simulink model "waypoint_follow"  (R2024a)
settings: Solver=VariableStepAuto  StartTime=0.0  StopTime=inf  RelTol=1e-3
libraries: rllib x1
settings Model: Creator=gaura  LastModifiedBy=gaura

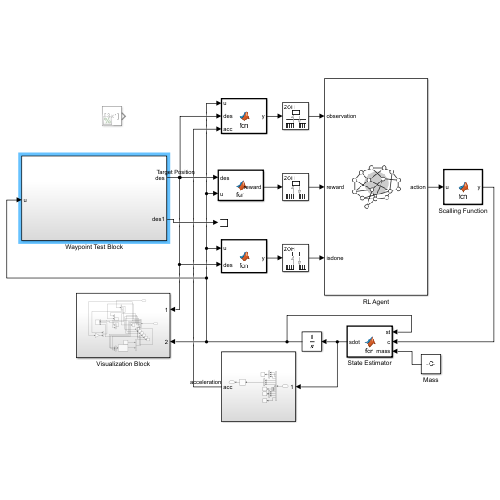
[thumbnail: Simulink's stored preview of the top-level diagram]
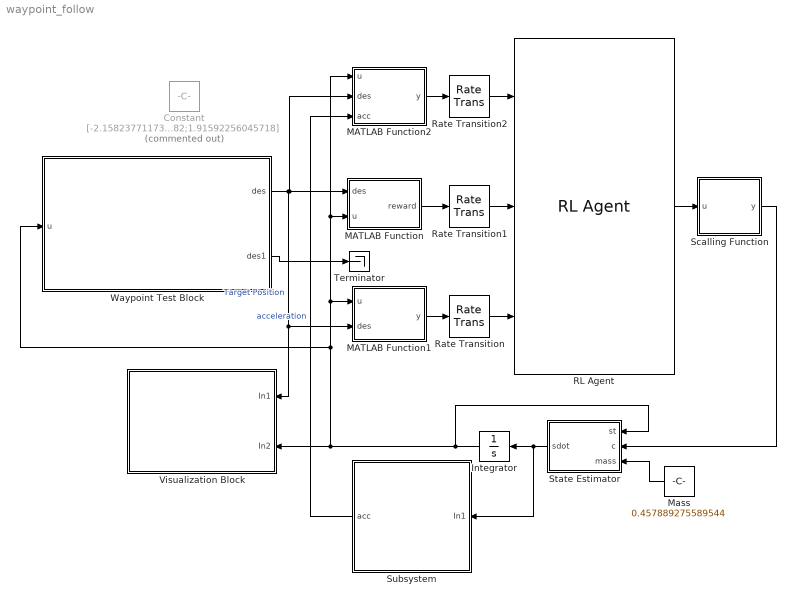
== system waypoint_follow ==
  Constant : Constant  Commented=on  Value=[-2.15823771173935;0.736471979161082;1.91592256045718]  SampleTime=-1
  Integrator : Integrator  InitialCondition=[2;-3;-1;0;0;0;0;0;0;0;0;0;0]
  MATLAB Function : MATLAB Function  TreatAsAtomicUnit=on
  MATLAB Function1 : MATLAB Function  TreatAsAtomicUnit=on
  MATLAB Function2 : MATLAB Function  TreatAsAtomicUnit=on
  Mass : Constant  Value=0.457889275589544  SampleTime=-1
  RL Agent : rllib/RL Agent  Agent=agent  ExternalActionAsInput=off  ProvideLastAction=off  ProvideCumRwd=off  TreatAsDirectFeedthrough=on  UseStrictObservationDataTypes=off
  Rate Transition : RateTransition
  Rate Transition1 : RateTransition
  Rate Transition2 : RateTransition
  Scalling Function : MATLAB Function  TreatAsAtomicUnit=on
  State Estimator : MATLAB Function  TreatAsAtomicUnit=on
  Subsystem : Subsystem
  Terminator : Terminator
  Visualization Block : Subsystem
  Waypoint Test Block : Subsystem
  wires:
  MATLAB Function/1(reward) -> Rate Transition1/1
  MATLAB Function1/1(y) -> Rate Transition/1
  MATLAB Function2/1(y) -> Rate Transition2/1
  RL Agent/1 -> Scalling Function/1(u)
  Scalling Function/1(y) -> State Estimator/2(c)
  State Estimator/1(sdot) -> Subsystem/1(In1), Integrator/1
  Integrator/1 -> MATLAB Function2/1(u), MATLAB Function/2(u), MATLAB Function1/1(u), Waypoint Test Block/1(u), Visualization Block/2(In2), State Estimator/1(st)
  Waypoint Test Block/1(des) -> MATLAB Function2/2(des), MATLAB Function/1(des), Visualization Block/1(In1), MATLAB Function1/2(des)  "Target Position"
  Rate Transition/1 -> RL Agent/3
  Rate Transition1/1 -> RL Agent/2
  Rate Transition2/1 -> RL Agent/1
  Mass/1 -> State Estimator/3(mass)
  Subsystem/1(acc) -> MATLAB Function2/3(acc)  "acceleration"
  Waypoint Test Block/2(des1) -> Terminator/1

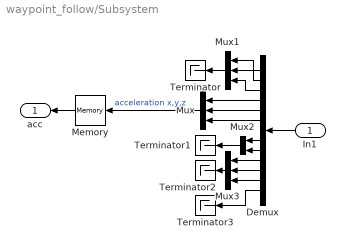
== system waypoint_follow/Subsystem ==
  In1 : Inport
  Demux : Demux  Outputs=13
  Memory : Memory  InitialCondition=[0;0;0]
  Mux : Mux  Inputs=3
  Mux1 : Mux  Inputs=3
  Mux2 : Mux  Inputs=2
  Mux3 : Mux  Inputs=3
  Terminator{,1..3} (4 alike) : Terminator
  acc : Outport
  wires:
  Demux/6 -> Mux/3
  Mux/1 -> Memory/1  "acceleration x,y,z"
  Memory/1 -> acc/1
  Demux/12 -> Mux3/3
  Demux/11 -> Mux3/2
  Demux/8 -> Mux2/1
  Demux/13 -> Terminator3/1
  Demux/3 -> Mux1/3
  Demux/4 -> Mux/1
  Demux/9 -> Mux2/2
  Demux/5 -> Mux/2
  Mux2/1 -> Terminator1/1
  Demux/10 -> Mux3/1
  Demux/1 -> Mux1/2
  Mux1/1 -> Terminator/1
  Demux/2 -> Mux1/1
  Mux3/1 -> Terminator2/1
  In1/1 -> Demux/1

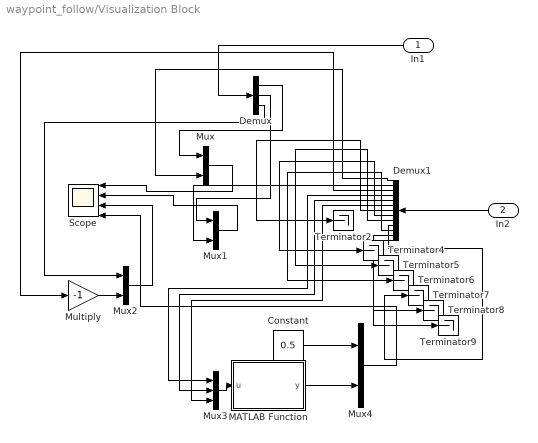
== system waypoint_follow/Visualization Block ==
  In1 : Inport
  In2 : Inport  Port=2
  Constant : Constant  Value=0.5  SampleTime=-1
  Demux : Demux  Outputs=3
  Demux1 : Demux  Outputs=13
  MATLAB Function : MATLAB Function  TreatAsAtomicUnit=on
  Multiply : Gain  Gain=-1
  Mux{,1..2,4} (4 alike) : Mux  Inputs=2
  Mux3 : Mux  Inputs=3
  Scope : Scope  NumInputPorts=4
  Terminator{2,4..9} (7 alike) : Terminator
  wires:
  Mux1/1 -> Scope/2
  Demux1/10 -> Terminator7/1
  Demux1/2 -> Mux1/2
  Demux1/1 -> Mux/2
  Demux1/13 -> Terminator9/1
  Demux1/6 -> Mux3/3
  Demux/2 -> Mux1/1
  Demux1/4 -> Mux3/1
  Demux1/7 -> Terminator2/1
  Mux/1 -> Scope/1
  Demux/3 -> Mux2/1
  Demux1/3 -> Multiply/1
  Demux1/9 -> Terminator5/1
  Demux1/11 -> Terminator6/1
  Demux1/8 -> Terminator4/1
  In2/1 -> Demux1/1
  Demux1/5 -> Mux3/2
  Demux1/12 -> Terminator8/1
  Mux2/1 -> Scope/3
  Demux/1 -> Mux/1
  In1/1 -> Demux/1
  Multiply/1 -> Mux2/2
  Mux3/1 -> MATLAB Function/1(u)
  MATLAB Function/1(y) -> Mux4/2
  Mux4/1 -> Scope/4
  Constant/1 -> Mux4/1

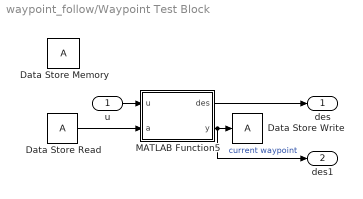
== system waypoint_follow/Waypoint Test Block ==
  u : Inport
  Data Store Memory : DataStoreMemory  WriteAfterWriteMsg=warning  InitialValue=1  ShowAdditionalParam=off
  Data Store Read : DataStoreRead  IndexOptions=Index vector (dialog)  Indices=1  OutputSizes=1
  Data Store Write : DataStoreWrite  IndexOptions=Index vector (dialog)  Indices=1  OutputSizes=1
  MATLAB Function5 : MATLAB Function  TreatAsAtomicUnit=on
  des : Outport
  des1 : Outport  Port=2
  wires:
  MATLAB Function5/2(y) -> des1/1, Data Store Write/1  "current waypoint"
  MATLAB Function5/1(des) -> des/1
  Data Store Read/1 -> MATLAB Function5/2(a)
  u/1 -> MATLAB Function5/1(u)

== matlab function waypoint_follow/MATLAB Function1 ==
  data: u input; y output; des input
function y = fcn(u,des)
    u(3) = -1 * u(3);
    % if norm(u(1:3) - des(1:3)) <= 0.01 && norm(u(4:6)) <= 0.05
    %     y = 1;
    % elseif u(3) >= 0 || norm(u(1:3) - des(1:3)) >= 10  % || norm(u(4:6)) > 1
    %     y = 1;
    % else
    %     y = 0;
    if norm(u(1:3) - des(1:3)) == 0.0 && norm(u(4:6)) < 0.01
        y = 1;
    elseif u(3) > 0% && norm(u(1:3) - des(1:3)) < 10 %&& norm(u(4:6)) <= 0.5
        y = 0;
    else
        y = 1;
    end
    % 
    % if norm(u(1:3) - des(1:3)) < 0.25
    %     y = 1;
    % else
    %     y = 0;
    % end

end

== matlab function waypoint_follow/MATLAB Function ==
  data: des input; u input; reward output
function reward  = fcn(des, u)
    u(3) = -1 * u(3);
    desired_pos = [des(1); des(2); des(3)];
    % desired_vel_moving = 0.5;  % Desired velocity while moving
    % desired_vel_stationary = 0;  % Desired velocity at the destination
    % ideal_value = 0.5;
    % deviation = 0.5;
    % vel = norm(u(4:6));
    % Compute the function value
    % r_v = max(0, 1 - abs(norm(u(4:6)) - ideal_value) / deviation);
    % weights for different component of reward
    w_p = 1;
    % w_v = 1;  % Weight for velocity reward
    
    % Extract values from observation
    p = [u(1); u(2); u(3)];
    v = [u(4); u(5); u(6)];
    % calculate indivisual component of reward
    % r_v = 2*(0.5 - abs(0.5 - norm(u(4:6))));
    % r_p = 1 - (norm(p-desired_pos)/10);
    r_p = w_p * (1 * exp(-1* norm(p-desired_pos)));
    % if norm(p - desired_pos) > 0.05
    %     % Drone is still moving towards the destination
    %     r_v = w_v * (1 * exp(-abs(norm(v) - desired_vel_moving)));  % Reward for maintaining velocity close to 0.5
    % else
    %     % Drone is at the destination, encourage stopping
    %     r_v = w_v * (1 * exp(-abs(norm(v) - desired_vel_stationary)));  % Reward for stopping (velocity near 0)
    % end
    % vel = norm(u(4:6));
    % if vel > 0.5
    %     r_v = exp(-5* abs(0.5 - vel));
    %     r_p = r_p * r_v;
    % end
    % r_p = 1 - (norm(p-desired_pos)/10);
    
    % dis = norm(p-desired_pos);
    % r_p = w_p * -1*dis ;
    % if norm(u(1:3) - des(1:3)) > 0.01
    %     % r_v = 1 - 2 * abs(0.5 - norm(u(4:6)));
    %     r_v = exp(-5* abs(0.5 - norm(u(4:6))));
    %     r_p = r_p * r_v;
    % end
    %     r_p = 1000;
    % elseif u(3) >= 0 || norm(u(1:3) - des(1:3)) >= 10
    %     r_p = -1000;
    % end
    % if vel > 0.45
    %     reward = r_p;
    % else
    %     reward = r_p;
    % end
    % Total reward
    % reward = r_p + r_v;
    reward = r_p;
    % if norm(u(1:3) - des(1:3)) < 0.05 && norm(u(4:6)) < 0.05
    %     reward = 100;
    % end
end

== matlab function waypoint_follow/MATLAB Function2 ==
  data: u input; y output; des input; acc input
function y = fcn(u,des,acc)
    u(3) = -1 * u(3);
    y = [u(3)/10;(u(1:3)-des(1:3))/10;u(4:6);(4*u(7:9))/pi;acc/10];
    % y = [u(3)/10;(u(1:3)-des(1:3))/10;u(4:6);(4*u(7:9))/pi];
end

== matlab function waypoint_follow/Scalling Function ==
  data: u input; y output
function y = fcn(u)
c1 = ((u(1) + 1) * (pi/2) / 2) - pi/4;
c2 = ((u(2) + 1) * (pi/2) / 2) - pi/4;
% c3 = ((u(3) + 1) * (pi/2) / 2) - pi/4;
% c4 = ((u(3) + 1) * (10) / 2) - 5;

% c1 = u(1) * 0.05;
% c2 = u(2) * 0.05;
% c3 = u(3) * 5;
c4 = (u(3) + 1) / 2;
c4 = c4 * 15;

% ax = c1;
% ay = c2;
% az = c3;
% 
% f = sqrt(ax^2 + ay^2 + az^2);
% % psi_des = rs_pos_des_msg.Data(4)*pi/180;
% psi_des = state(7);
% %phi_des = asin(-ay/f);
% %theta_des = asin(ax/(f*cos(phi_des)));
% ax2 =  ax*cos(psi_des) + ay*sin(psi_des);
% ay2 = -ax*sin(psi_des) + ay*cos(psi_des);
% phi_des = asin(-ay2/f);
% theta_des = asin(ax2/(f*cos(phi_des)));
% 
% %phi_des = asin((ax*sin(psi_des) - ay*cos(psi_des))/f);
% %theta_des = atan((-ay*sin(psi_des) + ax*cos(psi_des))/(0.65 + az));
% %theta_des = asin((ax*cos(psi_des) + ay*sin(psi_des))/(f*cos(phi_des)));
% 
% phi_des = max(-0.05,min(phi_des,0.05));
% theta_des = max(-0.05,min(theta_des,0.05));
% 
% az2 = (cos(phi_des)*sin(theta_des)*cos(psi_des) + sin(phi_des)*sin(psi_des))*ax + ...
%        (cos(phi_des)*sin(theta_des)*sin(psi_des) - sin(phi_des)*cos(psi_des))*ay + ...
%         (cos(phi_des)*cos(theta_des))*az;
% 
% T = az2;

y = [c1;c2;c4];
% y = [phi_des;theta_des;T];

== matlab function waypoint_follow/State Estimator ==
  data: st input; sdot output; c input; mass input
function sdot = fcn(st, c, mass)
    model = multirotor;
    model.Configuration.Mass = mass;
    s = state(model);
    s(1:13) = st;
    u = control(model);
    u.Roll = c(1);
    u.Pitch = c(2);
    % u.YawRate = c(3);
    u.Thrust = c(3);
    e = environment(model);
    sdot = derivative(model,s,u,e);
end

== matlab function waypoint_follow/Waypoint Test Block/MATLAB Function5 ==
  data: des output; u input; y output; a input
function [des,y] = fcn(u,a)
u(3) = -1 * u(3);

waypoints = [10,-6,5;0,-10,6;-10,-6,7;-12,0,8;0,9,9; 10,0,10];

if norm(u(1:3).' - waypoints(a,1:3)) < 0.11
    y = a+1;
else
    y=a;
end
if y > 6
    y = 6;
end
    
des = waypoints(y,1:3).';
end

== matlab function waypoint_follow/Visualization Block/MATLAB Function ==
  data: u input; y output
function y = fcn(u)

y = norm(u);
